simulink model "SignalGenerator"  (R2017b)
settings: Solver=VariableStepAuto  StartTime=0.0  StopTime=10.0  RelTol=1e-3
libraries: cstblocks x1, simulink x1, fl_lib x1
settings Model: Creator=k37107  LastModifiedBy=k37107

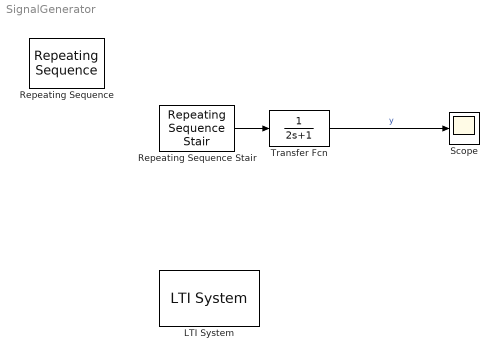
== system SignalGenerator ==
  LTI System : cstblocks/LTI System  sys=tf(1,[1 1])  IC=[]
  Repeating Sequence Stair : simulink/Sources/Repeating Sequence Stair  OutValues=[3 1 4 2 1].'  tsamp=-1  OutMin=[]  OutMax=[]  OutDataTypeStr=double  OutputDataTypeScalingMode=double  OutDataType=fixdt(0,8)  ConRadixGroup=Best Precision: Vector-wise  OutScaling=2^-12
  Repeating Sequence : fl_lib/Physical Signals/Sources/Repeating Sequence  y_init=0  offset=1 s  sig_type=1  durations=1 s  y_start=1  y_end=1
      settings: SourceProductName=Simscape  SourceProductBaseCode=SS
  Scope : Scope
  Transfer Fcn : TransferFcn  Denominator=[2 1]
  wires:
  Transfer Fcn/1 -> Scope/1  "y"
  Repeating Sequence Stair/1 -> Transfer Fcn/1
